simulink model "ModeShape_IEEE14"  (R2022b)
settings: Solver=FixedStepAuto  StartTime=0.0  StopTime=t_length  FixedStep=Ts  RelTol=1e-3
InitFcn:
  | if DEF_case==2  % 14 bus 8.8 Hz mode
  |     load('data_idq_all');
  |     idq_data_record = data_idq_all;
  |     load('data_vdq_all');
  |     vdq_data_record = data_vdq_all;
  |     ModeSel = 151;
  |     pll_pid = [50 20 1];
  |     Tpll_d = Ts*10;
  |     Tpll_s = Ts*10;
  |     fpll_c = 4;
  |     t_length = 15;
  | end
  | 
  | 
  | if DEF_case==3 %14 bus 1.5 Hz mode
  |     load('data_idq_all_case2');
  |     idq_data_record = data_idq_all_case2;
  |     load('data_vdq_all_case2');
  |     vdq_data_record = data_vdq_all_case2;
  |     ModeSel = 202;
  |     pll_pid = [3 0.8 0.1];
  |     Tpll_d = Ts*10;
  |     Tpll_s = Ts*10;
  |     fpll_c = 1;
  |     t_length = 60;
  | end
  | run Mode_Right_Eig.m;
values from neighbouring files (symbols this model uses):
  freq_sel = imag(Mode_Hz)    [Mode_Right_Eig.m]
  Mode_Rad = D(ModeSel, ModeSel)    [Mode_Right_Eig.m]
  Phi_vec_trim = Phi_vec_trim.'    [Mode_Right_Eig.m]
  Psi_vec_trim = Psi_vec_trim.'    [Mode_Right_Eig.m]
undefined symbols (not defined in the file or in its folder): DEF_case, Ts
libraries: eeGeneralControl x6, spsPLLLib x1
settings Model: Creator=y_zhu  LastModifiedBy=yz34218

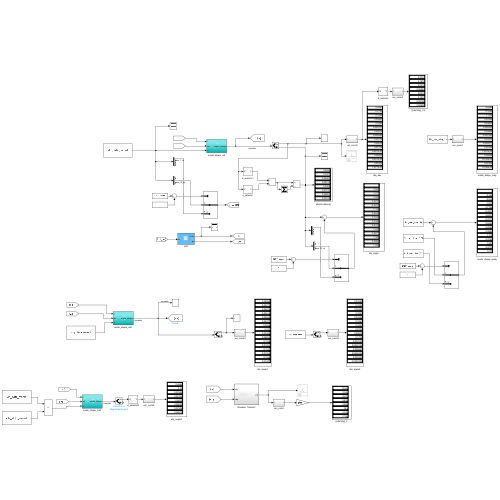
[thumbnail: Simulink's stored preview of the top-level diagram]
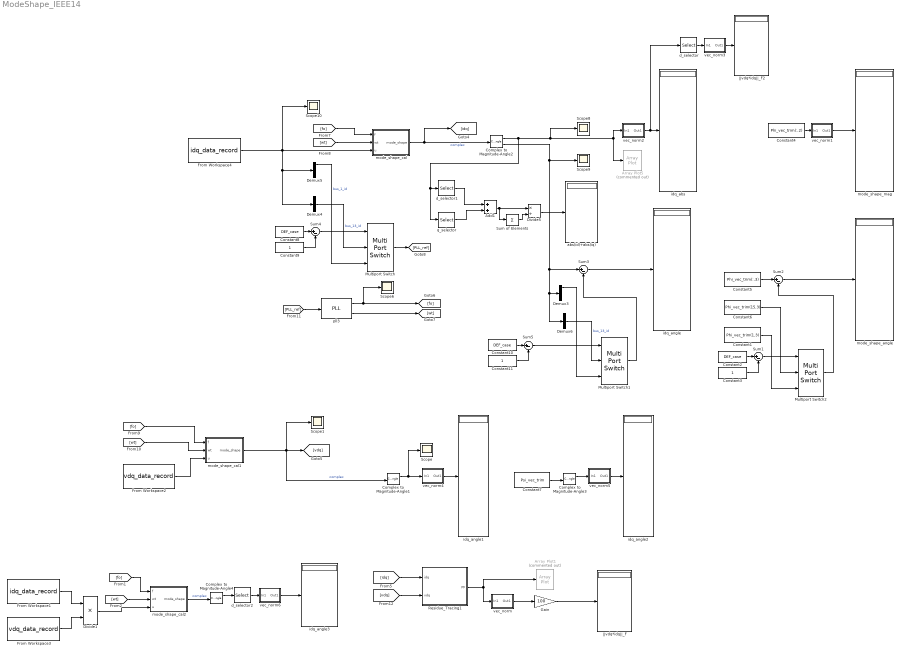
== system ModeShape_IEEE14 ==
  Add1 : Sum
  Array Plot1 : ArrayPlot  Commented=on  WindowPosition=[-1902.000000,100.000000,800.000000,500.000000,]  ScopeFrameLocation=window  YLimits=[-0.0014,0.0131]
  Array Plot5 : ArrayPlot  Commented=on  WindowPosition=[-1889.000000,191.000000,800.000000,500.000000,]  ScopeFrameLocation=window  YLimits=[-0.0014,0.0131]
  Complex to Magnitude-Angle{1..4} (4 alike) : ComplexToMagnitudeAngle
  Constant1 : Constant  Value=Phi_vec_trim(1,3)
  Constant10 : Constant  Value=DEF_case
  Constant11 : Constant
  Constant2 : Constant  Value=DEF_case
  Constant3 : Constant
  Constant4 : Constant  Value=Phi_vec_trim(:,2)
  Constant5 : Constant  Value=Phi_vec_trim(:,3)
  Constant6 : Constant  Value=Phi_vec_trim(15,3)
  Constant7 : Constant  Value=Psi_vec_trim
  Constant8 : Constant  Value=DEF_case
  Constant9 : Constant
  Demux3 : Demux  Outputs=[1,11,1,3]
  Demux4 : Demux  Outputs=[14,1,1]
  Demux5 : Demux  Outputs=[1,11,1,3]
  Demux6 : Demux  Outputs=[14,1,1]
  Divide1 : Product  Inputs=**
  Divide5 : Product  Inputs=*/
  From Workspace1 : FromWorkspace  VariableName=idq_data_record
  From Workspace2 : FromWorkspace  VariableName=vdq_data_record
  From Workspace3 : FromWorkspace  VariableName=vdq_data_record
  From Workspace4 : FromWorkspace  VariableName=idq_data_record
  Gain : Gain  Gain=100
  Multiport Switch : MultiPortSwitch  Inputs=2  SaturateOnIntegerOverflow=off  InputSameDT=off
  Multiport Switch1 : MultiPortSwitch  Inputs=2  SaturateOnIntegerOverflow=off  InputSameDT=off
  Multiport Switch2 : MultiPortSwitch  Inputs=2  SaturateOnIntegerOverflow=off  InputSameDT=off
  Residue_Tracing1 : Subsystem
  Scope{,1,6,8..10} (6 alike) : Scope
  Sum of Elements : Sum  Inputs=+
  Sum{1..5} (5 alike) : Sum  Inputs=|+-
  abs(id)+abs(iq) : Display
  d_selector : Selector  InputPortWidth=length(Phi_vec_trim)  IndexOptions=Index vector (dialog)  Indices=[1:2:length(Phi_vec_trim)]  OutputSizes=1
  d_selector1 : Selector  InputPortWidth=length(Phi_vec_trim)  IndexOptions=Index vector (dialog)  Indices=[1:2:length(Phi_vec_trim)]  OutputSizes=1
  d_selector2 : Selector  InputPortWidth=length(Phi_vec_trim)  IndexOptions=Index vector (dialog)  Indices=[1:2:length(Phi_vec_trim)]  OutputSizes=1
  idq_abs : Display
  idq_angle{,1..3} (4 alike) : Display
  mode_shape_angle : Display
  mode_shape_cal : Subsystem
  mode_shape_cal1 : Subsystem
  mode_shape_cal2 : Subsystem
  mode_shape_mag : Display
  pll3 : spsPLLLib/PLL  Fmin=freq_sel/2  Par_Init=[0, freq_sel]  ParK=pll_pid  TcD=Tpll_d  MaxRateChangeFreq=1  FilterCutOffFreq=fpll_c  Ts=Tpll_s  AGC=on
      settings: LibrarySourceBlock=sps_lib/Control/PLL
  q_selector : Selector  InputPortWidth=length(Phi_vec_trim)  IndexOptions=Index vector (dialog)  Indices=[2:2:length(Phi_vec_trim)]  OutputSizes=1
  vec_norm : Subsystem
  vec_norm1 : Subsystem
  vec_norm2 : Subsystem
  vec_norm3 : Subsystem
  vec_norm4 : Subsystem
  vec_norm5 : Subsystem
  vec_norm6 : Subsystem
  ||vdq*idq||_F : Display
  ||vdq*idq||_F2 : Display
  wires:
  q_selector/1 -> Add1/2
  Residue_Tracing1/1(PF) -> Array Plot1/1, vec_norm/1(In1)
  [idq] -> Residue_Tracing1/1(idq)
  d_selector1/1 -> Add1/1
  Demux3/1 -> Multiport Switch1/3
  mode_shape_cal/1(mode_shape) -> Complex to Magnitude-Angle2/1, [idq]  "complex"
  Complex to Magnitude-Angle2/1 -> q_selector/1, d_selector1/1, Array Plot5/1, vec_norm2/1(In1), Scope8/1
  Constant5/1 -> Sum2/1
  [wt] -> mode_shape_cal/2(wt)
  [fo] -> mode_shape_cal/1(f)
  Complex to Magnitude-Angle2/2 -> Scope9/1, Demux6/1, Demux3/1, Sum3/1
  [PLL_ref] -> pll3/1
  Constant4/1 -> vec_norm1/1(In1)
  Sum3/1 -> idq_angle/1
  Divide5/1 -> abs(id)+abs(iq)/1
  Add1/1 -> Divide5/1, Sum of Elements/1
  [wt] -> mode_shape_cal1/2(wt)
  Sum2/1 -> mode_shape_angle/1
  Sum of Elements/1 -> Divide5/2
  From Workspace2/1 -> mode_shape_cal1/3(u)
  Gain/1 -> ||vdq*idq||_F/1
  vec_norm/1(Out1) -> Gain/1
  [vdq] -> Residue_Tracing1/2(vdq)
  [fo] -> mode_shape_cal1/1(f)
  From Workspace4/1 -> Scope10/1, Demux4/1, Demux5/1, mode_shape_cal/3(u)
  Constant8/1 -> Sum4/1
  Constant9/1 -> Sum4/2
  Sum4/1 -> Multiport Switch/1
  Multiport Switch/1 -> [PLL_ref]
  Constant11/1 -> Sum5/2
  Sum5/1 -> Multiport Switch1/1
  Constant10/1 -> Sum5/1
  Demux6/2 -> Multiport Switch1/2  "bus_13_id"
  Multiport Switch1/1 -> Sum3/2
  Demux4/2 -> Multiport Switch/2  "bus_13_id"
  pll3/1 -> Scope6/1, [fo]
  pll3/2 -> [wt]
  Demux5/1 -> Multiport Switch/3  "bus_1_id"
  Constant3/1 -> Sum1/2
  Sum1/1 -> Multiport Switch2/1
  Constant2/1 -> Sum1/1
  Constant6/1 -> Multiport Switch2/2
  Constant1/1 -> Multiport Switch2/3
  Multiport Switch2/1 -> Sum2/2
  vec_norm1/1(Out1) -> mode_shape_mag/1
  vec_norm2/1(Out1) -> d_selector/1, idq_abs/1
  d_selector/1 -> vec_norm3/1(In1)
  vec_norm3/1(Out1) -> ||vdq*idq||_F2/1
  vec_norm5/1(Out1) -> idq_angle2/1
  Complex to Magnitude-Angle1/1 -> Scope/1, vec_norm4/1(In1)
  vec_norm4/1(Out1) -> idq_angle1/1
  Constant7/1 -> Complex to Magnitude-Angle3/1
  Complex to Magnitude-Angle3/1 -> vec_norm5/1(In1)
  mode_shape_cal1/1(mode_shape) -> Scope1/1, Complex to Magnitude-Angle1/1, [vdq]  "complex"
  From Workspace1/1 -> Divide1/1
  From Workspace3/1 -> Divide1/2
  Divide1/1 -> mode_shape_cal2/3(u)
  [fo] -> mode_shape_cal2/1(f)
  [wt] -> mode_shape_cal2/2(wt)
  mode_shape_cal2/1(mode_shape) -> Complex to Magnitude-Angle4/1  "complex"
  Complex to Magnitude-Angle4/1 -> d_selector2/1
  vec_norm6/1(Out1) -> idq_angle3/1
  d_selector2/1 -> vec_norm6/1(In1)

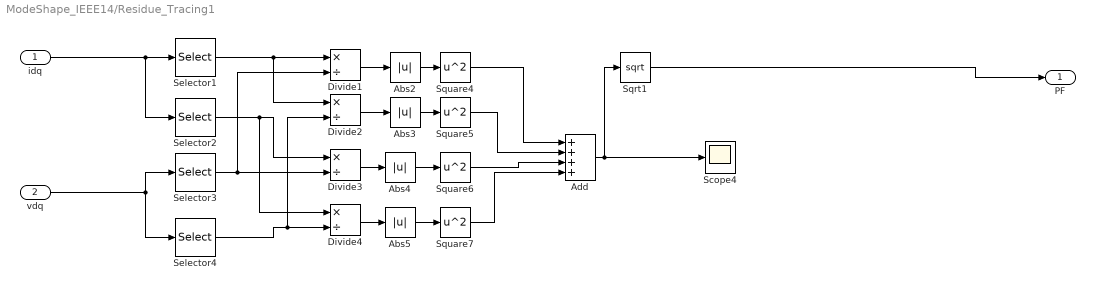
== system ModeShape_IEEE14/Residue_Tracing1 ==
  idq : Inport
  vdq : Inport  Port=2
  Abs{2..5} (4 alike) : Abs  SaturateOnIntegerOverflow=off
  Add : Sum  Inputs=++++
  Divide{1..4} (4 alike) : Product  Inputs=*/
  Scope4 : Scope
  Selector1 : Selector  InputPortWidth=16  IndexOptions=Index vector (dialog)  Indices=[1:2:15]  OutputSizes=1
  Selector2 : Selector  InputPortWidth=16  IndexOptions=Index vector (dialog)  Indices=[2:2:16]  OutputSizes=1
  Selector3 : Selector  InputPortWidth=16  IndexOptions=Index vector (dialog)  Indices=[1:2:15]  OutputSizes=1
  Selector4 : Selector  InputPortWidth=16  IndexOptions=Index vector (dialog)  Indices=[2:2:16]  OutputSizes=1
  Sqrt1 : Sqrt
  Square{4..7} (4 alike) : Math  Operator=square
  PF : Outport
  wires:
  Selector2/1 -> Divide4/1, Divide3/1
  Square6/1 -> Add/3
  Selector4/1 -> Divide2/2, Divide4/2
  Divide1/1 -> Abs2/1
  vdq/1 -> Selector4/1, Selector3/1
  idq/1 -> Selector2/1, Selector1/1
  Selector1/1 -> Divide2/1, Divide1/1
  Abs5/1 -> Square7/1
  Divide2/1 -> Abs3/1
  Selector3/1 -> Divide3/2, Divide1/2
  Divide4/1 -> Abs5/1
  Divide3/1 -> Abs4/1
  Abs2/1 -> Square4/1
  Add/1 -> Scope4/1, Sqrt1/1
  Abs4/1 -> Square6/1
  Abs3/1 -> Square5/1
  Square4/1 -> Add/1
  Square5/1 -> Add/2
  Square7/1 -> Add/4
  Sqrt1/1 -> PF/1

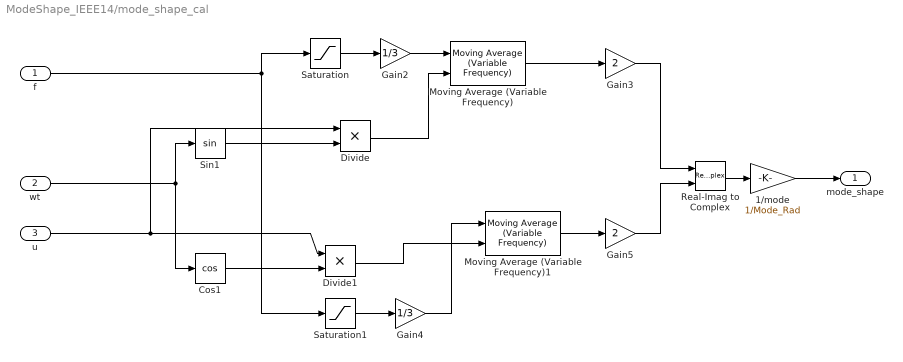
== system ModeShape_IEEE14/mode_shape_cal ==
  f : Inport
  wt : Inport  Port=2
  u : Inport  Port=3
  1/mode : Gain  Gain=1/Mode_Rad
  Cos1 : Trigonometry  Operator=cos
  Divide : Product  Inputs=**
  Divide1 : Product  Inputs=**
  Gain2 : Gain  Gain=1/3
  Gain3 : Gain  Gain=2
  Gain4 : Gain  Gain=1/3
  Gain5 : Gain  Gain=2
  Moving Average (Variable Frequency) : eeGeneralControl/Moving Average (Variable Frequency)  VariantControl=Variant1  LabelModeActiveChoice=Discrete  f0=freq_sel/3  fmin=0.1  x0=0  BufferSize=8192  Ts=Ts*100
      settings: LibrarySourceBlock=|
      | ee_sl_lib/General Control/Moving Average
      | (Variable Frequency)
  Moving Average (Variable Frequency)1 : eeGeneralControl/Moving Average (Variable Frequency)  VariantControl=Variant1  LabelModeActiveChoice=Discrete  f0=freq_sel/3  fmin=0.1  x0=0  BufferSize=8192  Ts=Ts*100
      settings: LibrarySourceBlock=|
      | ee_sl_lib/General Control/Moving Average
      | (Variable Frequency)
  Real-Imag to Complex : RealImagToComplex
  Saturation : Saturate  UpperLimit=freq_sel+0.5  LowerLimit=freq_sel-0.5
  Saturation1 : Saturate  UpperLimit=freq_sel+0.5  LowerLimit=freq_sel-0.5
  Sin1 : Trigonometry
  mode_shape : Outport
  wires:
  wt/1 -> Cos1/1, Sin1/1
  Divide1/1 -> Moving Average (Variable Frequency)1/2
  Cos1/1 -> Divide1/2
  Saturation1/1 -> Gain4/1
  Moving Average (Variable Frequency)1/1 -> Gain5/1
  Saturation/1 -> Gain2/1
  Gain2/1 -> Moving Average (Variable Frequency)/1
  f/1 -> Saturation1/1, Saturation/1
  Gain4/1 -> Moving Average (Variable Frequency)1/1
  Divide/1 -> Moving Average (Variable Frequency)/2
  Real-Imag to Complex/1 -> 1/mode/1
  Gain3/1 -> Real-Imag to Complex/1
  Gain5/1 -> Real-Imag to Complex/2
  u/1 -> Divide1/1, Divide/1
  Moving Average (Variable Frequency)/1 -> Gain3/1
  Sin1/1 -> Divide/2
  1/mode/1 -> mode_shape/1

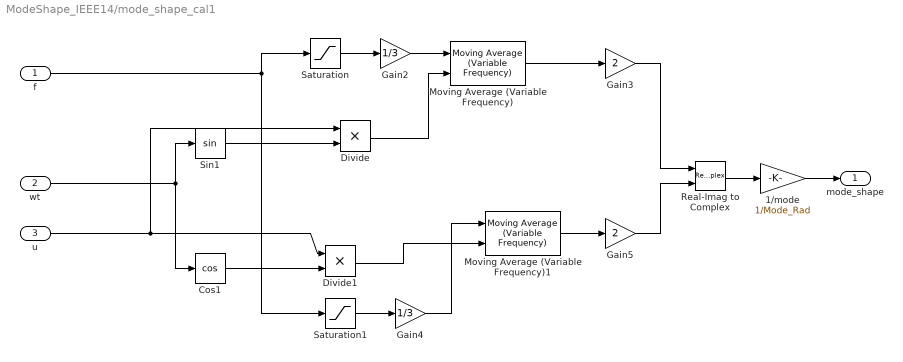
== system ModeShape_IEEE14/mode_shape_cal1 ==
  f : Inport
  wt : Inport  Port=2
  u : Inport  Port=3
  1/mode : Gain  Gain=1/Mode_Rad
  Cos1 : Trigonometry  Operator=cos
  Divide : Product  Inputs=**
  Divide1 : Product  Inputs=**
  Gain2 : Gain  Gain=1/3
  Gain3 : Gain  Gain=2
  Gain4 : Gain  Gain=1/3
  Gain5 : Gain  Gain=2
  Moving Average (Variable Frequency) : eeGeneralControl/Moving Average (Variable Frequency)  VariantControl=Variant1  LabelModeActiveChoice=Discrete  f0=freq_sel/3  fmin=0.1  x0=0  BufferSize=8192  Ts=Ts*100
      settings: LibrarySourceBlock=|
      | ee_sl_lib/General Control/Moving Average
      | (Variable Frequency)
  Moving Average (Variable Frequency)1 : eeGeneralControl/Moving Average (Variable Frequency)  VariantControl=Variant1  LabelModeActiveChoice=Discrete  f0=freq_sel/3  fmin=0.1  x0=0  BufferSize=8192  Ts=Ts*100
      settings: LibrarySourceBlock=|
      | ee_sl_lib/General Control/Moving Average
      | (Variable Frequency)
  Real-Imag to Complex : RealImagToComplex
  Saturation : Saturate  UpperLimit=freq_sel+0.5  LowerLimit=freq_sel-0.5
  Saturation1 : Saturate  UpperLimit=freq_sel+0.5  LowerLimit=freq_sel-0.5
  Sin1 : Trigonometry
  mode_shape : Outport
  wires:
  wt/1 -> Cos1/1, Sin1/1
  Divide1/1 -> Moving Average (Variable Frequency)1/2
  Cos1/1 -> Divide1/2
  Saturation1/1 -> Gain4/1
  Moving Average (Variable Frequency)1/1 -> Gain5/1
  Saturation/1 -> Gain2/1
  Gain2/1 -> Moving Average (Variable Frequency)/1
  f/1 -> Saturation1/1, Saturation/1
  Gain4/1 -> Moving Average (Variable Frequency)1/1
  Divide/1 -> Moving Average (Variable Frequency)/2
  Gain3/1 -> Real-Imag to Complex/1
  Gain5/1 -> Real-Imag to Complex/2
  u/1 -> Divide1/1, Divide/1
  Moving Average (Variable Frequency)/1 -> Gain3/1
  Sin1/1 -> Divide/2
  Real-Imag to Complex/1 -> 1/mode/1
  1/mode/1 -> mode_shape/1

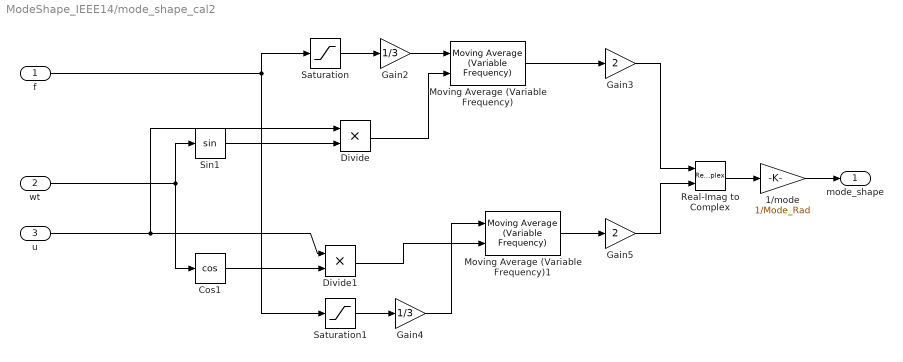
== system ModeShape_IEEE14/mode_shape_cal2 ==
  f : Inport
  wt : Inport  Port=2
  u : Inport  Port=3
  1/mode : Gain  Gain=1/Mode_Rad
  Cos1 : Trigonometry  Operator=cos
  Divide : Product  Inputs=**
  Divide1 : Product  Inputs=**
  Gain2 : Gain  Gain=1/3
  Gain3 : Gain  Gain=2
  Gain4 : Gain  Gain=1/3
  Gain5 : Gain  Gain=2
  Moving Average (Variable Frequency) : eeGeneralControl/Moving Average (Variable Frequency)  VariantControl=Variant1  LabelModeActiveChoice=Discrete  f0=freq_sel/3  fmin=0.1  x0=0  BufferSize=8192  Ts=Ts*100
      settings: LibrarySourceBlock=|
      | ee_sl_lib/General Control/Moving Average
      | (Variable Frequency)
  Moving Average (Variable Frequency)1 : eeGeneralControl/Moving Average (Variable Frequency)  VariantControl=Variant1  LabelModeActiveChoice=Discrete  f0=freq_sel/3  fmin=0.1  x0=0  BufferSize=8192  Ts=Ts*100
      settings: LibrarySourceBlock=|
      | ee_sl_lib/General Control/Moving Average
      | (Variable Frequency)
  Real-Imag to Complex : RealImagToComplex
  Saturation : Saturate  UpperLimit=freq_sel+0.5  LowerLimit=freq_sel-0.5
  Saturation1 : Saturate  UpperLimit=freq_sel+0.5  LowerLimit=freq_sel-0.5
  Sin1 : Trigonometry
  mode_shape : Outport
  wires:
  wt/1 -> Cos1/1, Sin1/1
  Divide1/1 -> Moving Average (Variable Frequency)1/2
  Cos1/1 -> Divide1/2
  Saturation1/1 -> Gain4/1
  Moving Average (Variable Frequency)1/1 -> Gain5/1
  Saturation/1 -> Gain2/1
  Gain2/1 -> Moving Average (Variable Frequency)/1
  f/1 -> Saturation1/1, Saturation/1
  Gain4/1 -> Moving Average (Variable Frequency)1/1
  Divide/1 -> Moving Average (Variable Frequency)/2
  Gain3/1 -> Real-Imag to Complex/1
  Gain5/1 -> Real-Imag to Complex/2
  u/1 -> Divide1/1, Divide/1
  Moving Average (Variable Frequency)/1 -> Gain3/1
  Sin1/1 -> Divide/2
  Real-Imag to Complex/1 -> 1/mode/1
  1/mode/1 -> mode_shape/1

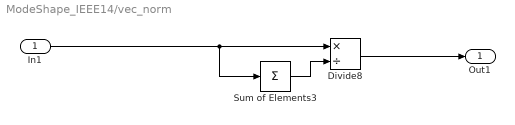
== system ModeShape_IEEE14/vec_norm ==
  In1 : Inport
  Divide8 : Product  Inputs=*/
  Sum of Elements3 : Sum  Inputs=+
  Out1 : Outport
  wires:
  Sum of Elements3/1 -> Divide8/2
  In1/1 -> Sum of Elements3/1, Divide8/1
  Divide8/1 -> Out1/1

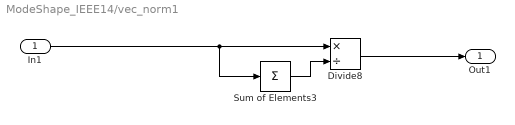
== system ModeShape_IEEE14/vec_norm1 ==
  In1 : Inport
  Divide8 : Product  Inputs=*/
  Sum of Elements3 : Sum  Inputs=+
  Out1 : Outport
  wires:
  Sum of Elements3/1 -> Divide8/2
  In1/1 -> Sum of Elements3/1, Divide8/1
  Divide8/1 -> Out1/1

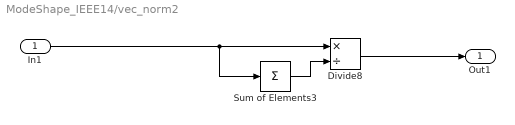
== system ModeShape_IEEE14/vec_norm2 ==
  In1 : Inport
  Divide8 : Product  Inputs=*/
  Sum of Elements3 : Sum  Inputs=+
  Out1 : Outport
  wires:
  Sum of Elements3/1 -> Divide8/2
  In1/1 -> Sum of Elements3/1, Divide8/1
  Divide8/1 -> Out1/1

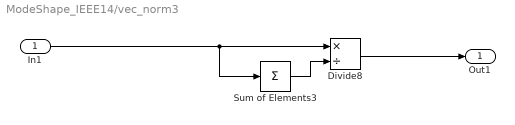
== system ModeShape_IEEE14/vec_norm3 ==
  In1 : Inport
  Divide8 : Product  Inputs=*/
  Sum of Elements3 : Sum  Inputs=+
  Out1 : Outport
  wires:
  Sum of Elements3/1 -> Divide8/2
  In1/1 -> Sum of Elements3/1, Divide8/1
  Divide8/1 -> Out1/1

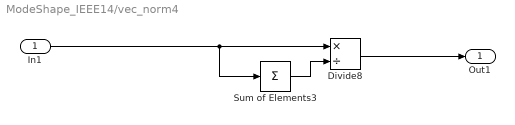
== system ModeShape_IEEE14/vec_norm4 ==
  In1 : Inport
  Divide8 : Product  Inputs=*/
  Sum of Elements3 : Sum  Inputs=+
  Out1 : Outport
  wires:
  Sum of Elements3/1 -> Divide8/2
  In1/1 -> Sum of Elements3/1, Divide8/1
  Divide8/1 -> Out1/1

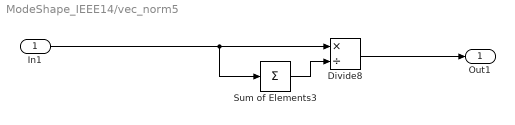
== system ModeShape_IEEE14/vec_norm5 ==
  In1 : Inport
  Divide8 : Product  Inputs=*/
  Sum of Elements3 : Sum  Inputs=+
  Out1 : Outport
  wires:
  Sum of Elements3/1 -> Divide8/2
  In1/1 -> Sum of Elements3/1, Divide8/1
  Divide8/1 -> Out1/1

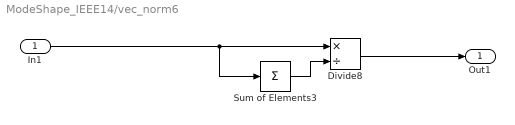
== system ModeShape_IEEE14/vec_norm6 ==
  In1 : Inport
  Divide8 : Product  Inputs=*/
  Sum of Elements3 : Sum  Inputs=+
  Out1 : Outport
  wires:
  Sum of Elements3/1 -> Divide8/2
  In1/1 -> Sum of Elements3/1, Divide8/1
  Divide8/1 -> Out1/1
